simulink model "duffing_sim"  (R2019b)
settings: Solver=FixedStepAuto  StartTime=0.0  StopTime=t_end  FixedStep=dt  MaxStep=.1  RelTol=1e-3
settings Model: Creator=enrique.babio  LastModifiedBy=enrique.babio
settings DataIOCC: ExternalInput=getinputstruct(opTrim)  InitialState=getstatestruct(opTrim)  SaveState=on

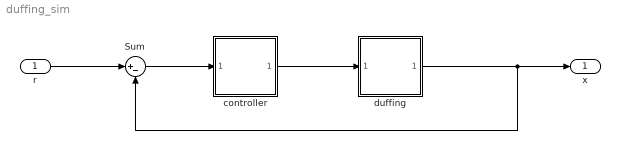
== system duffing_sim ==
  r : Inport
  Sum : Sum  Inputs=|+-
  controller : Subsystem  ReferencedSubsystem=controller
  duffing : Subsystem  ReferencedSubsystem=duffing
  x : Outport
  wires:
  duffing/1 -> Sum/2, x/1
  controller/1 -> duffing/1
  r/1 -> Sum/1
  Sum/1 -> controller/1
